simulink model "ModelDemopalooza"  (R2022b)
settings: Solver=FixedStepDiscrete  StartTime=0.0  StopTime=1  RelTol=1e-3  EnableMultiTasking=on
InitFcn:
  | % Initialize model
  | run(['ModelInit.m']);
  | 
  | % load library data
  | GainLibrary_data;
StartFcn:
  | % make sure all the simulated RTC requests are found
  | %RTC_SIM_OBJ.ValidateREQs();
model workspace (MAT data in the model file):
  PreampVolumeTable_Idx : Simulink.Signal (value not decoded)
  Range : Simulink.Signal (value not decoded)
  Table_Idx : Simulink.Signal (value not decoded)
undefined symbols (not defined in the file): Config, Ifir, IFIR, MedusaConfig, MuteRamper, MuteRamperBtc, numAudioIn, preAmp, Row, sys_defs, VLSConfig
libraries: FeaturePath x22, TuneVar x17, RTC x9, MedusaDelays x9, dspindex x5, TOP x5, SampleRateConverter x4, EdgePorts x2, PooliirLib x2, MedusaCaeEnable x2, FIREven x2, VLSGains x2
(part 4 of 4)

== matlab function ModelDemopalooza/PostProcess/Reset/MATLAB Function ==
  events: trigger input FUNCTION_CALL_EVENT
function fcn()

if coder.target('Rtw')
    coder.ceval('Model_Target_PostProcess_initialize');
    coder.ceval('Model_Target_PostProcess_Start');
    coder.ceval('Model_Target_PostProcess_Init');
end

== matlab function ModelDemopalooza/PreAmp/DecRate/Medusa5H1/MedusaHoligram/Medusa5H1 Part 4/On/Headrest Comp EQ/Delay Line Update ==
  data: u input; y output; delayChans input; inputMapping input; states data_store_memory; stateIndex data_store_memory; fixedDelayLength parameter
function y = delayLineUpdate(u, delayChans, inputMapping, fixedDelayLength)

% Note: This block only reads 'states' to get the delayed samples. A
% separate function is responsible for writing to 'states' to update the 
% delay line Data Store Memory. Thus it is important to ensure all DSM  
% write happens before DSM read.
%
% This is different from pooldelay, as the delay for ALL channel is
% intentionally set to be the max amount to allow for 'double' sharing
% between FIR filter and delay buffer.

global states;
global stateIndex; 

numOutput = numel(delayChans);
[frameSize, numChannelIn] = size(u);
y = single(zeros(frameSize, numOutput));
delayChans = int32(delayChans);

% Write incoming input to delay line
writeIdx = stateIndex;
for sample = 1:frameSize
    for i = 1:numChannelIn
        states(writeIdx+1,i) = u(sample, i); % add 1 for Matlab indexing
    end
    writeIdx = circindex(writeIdx, int32(1), fixedDelayLength);
end
stateIndex = writeIdx;

% Read out values from delay line
for i = 1:numOutput
    inputIdx = inputMapping(i);  % which input to delay
    delay = delayChans(i);       % delay amount
    offset = - (delay + frameSize); % offset from start index
    readIdx = circindex(stateIndex, offset, fixedDelayLength);
    
    for sample = 1:frameSize
        y(sample, i) = states(readIdx+1, inputIdx+1); % add 1 for Matlab indexing
        readIdx = circindex(readIdx, int32(1), fixedDelayLength);
    end
end
